simulink model "e8_1_sim"  (R2017b)
settings: Solver=ode4  StartTime=0.0  StopTime=30  FixedStep=0.001  RelTol=1e-3
values from neighbouring files (symbols this model uses):
  DEG2RAD = 0.0174533    [Init_control.m]
  Kd_PITCH_AngleRate = 0.001    [Init_control.m]
  Kd_ROLL_AngleRate = 0.001    [Init_control.m]
  Kd_YAW_AngleRate = 0.00    (= 0)    [Init_control.m]
  Ki_PITCH_AngleRate = 0.02    [Init_control.m]
  Ki_ROLL_AngleRate = 0.02    [Init_control.m]
  Ki_YAW_AngleRate = 0.01    [Init_control.m]
  Kp_PITCH_ANGLE = 6.5    [Init_control.m]
  Kp_PITCH_AngleRate = 0.1    [Init_control.m]
  Kp_ROLL_ANGLE = 6.5    [Init_control.m]
  Kp_ROLL_AngleRate = 0.1    [Init_control.m]
  Kp_YAW_ANGLE = 3    [Init_control.m]
  Kp_YAW_AngleRate = 0.5    [Init_control.m]
  Kpxp = 1.0    (= 1)    [Init_control.m]
  Kpyp = 1.0    (= 1)    [Init_control.m]
  Kpzp = 4.0    (= 4)    [Init_control.m]
  Kvxd = 0.01    [Init_control.m]
  Kvxi = 0.1    [Init_control.m]
  Kvxp = 3.0    (= 3)    [Init_control.m]
  Kvyd = 0.01    [Init_control.m]
  Kvyi = 0.1    [Init_control.m]
  Kvyp = 3.0    (= 3)    [Init_control.m]
  Kvzd = 0.005    [Init_control.m]
  Kvzi = 0.01    [Init_control.m]
  Kvzp = 0.45    [Init_control.m]
  MAX_CONTROL_ANGLE_NAV_PITCH = 15    [Init_control.m]
  MAX_CONTROL_ANGLE_NAV_ROLL = 15    [Init_control.m]
  MAX_CONTROL_ANGLE_PITCH = 35    [Init_control.m]
  MAX_CONTROL_ANGLE_RATE_PITCH = 220    [Init_control.m]
  MAX_CONTROL_ANGLE_RATE_ROLL = 220    [Init_control.m]
  MAX_CONTROL_ANGLE_RATE_Y = 200    [Init_control.m]
  MAX_CONTROL_ANGLE_ROLL = 35    [Init_control.m]
  MAX_CONTROL_VELOCITY_XY = 5    [Init_control.m]
  MAX_CONTROL_VELOCITY_Z = 3    [Init_control.m]
  Saturation_I_ah = 3.43    [Init_control.m]
  Saturation_I_az = 5    [Init_control.m]
  Saturation_I_RP_Max = 0.3    [Init_control.m]
  Saturation_I_RP_Min = -0.3    [Init_control.m]
  Saturation_I_Y_Max = 0.2    [Init_control.m]
  Saturation_I_Y_Min = -0.2    [Init_control.m]
  THR_HOVER = 0.609    [Init_control.m]
undefined symbols (not defined in the file or in its folder): DiscIntNeverNeededParam, earthRadius, KiRollAttitude, ModelInit_AngEuler, ModelInit_PosE, ModelInit_Rads, ModelInit_RateB, ModelInit_VelB, ModelParam_envGravityAcc, ModelParam_motorCr, ModelParam_motorJm, ModelParam_motorT, ModelParam_motorWb, ModelParam_rotorCm, ModelParam_rotorCt, ModelParam_uavCd, ModelParam_uavJ, ModelParam_uavMass, ModelParam_uavR, Receive, Send
libraries: simulink x10, aerolibfltsims x3, sharedutil x2, aerolibanimutils x1
(part 2 of 2)

== matlab function e8_1_sim/Control System/InputConditioning/deadzone2 ==
  data: u input; y output
function y = fcn(u)
%Function description:
%  Control the range of the remote control input from RCMin to RCMax, and set
%  a dead zone with a dead zone size of ±deadZone,the output y is
%  normalized to 0~1.You can get the RC calibration parameters in QGC.
RCMin = 1100;
RCMax = 1900;
RCMid = (RCMin + RCMax)/2;
deadZoneRate = 0.05;
deadZone = deadZoneRate*(RCMax - RCMin);
k = 1/(RCMax - RCMid - deadZone);
%Limiting
if(u < RCMin)
    u = RCMin;
elseif(u > RCMax)
    u = RCMax;
end
%dead zone and normalize
 if(u > RCMid + deadZone)
    y = (u-RCMid - deadZone)*k;
 elseif(u < RCMid - deadZone)
     y = (u - RCMid + deadZone)*k;
 else
     y = 0;
 end

 end

== matlab function e8_1_sim/Control System/Subsystem/AttitudeControl/yawAngle_d/MATLAB Function1 ==
  settings: updateMethod=DISCRETE
  data: yaw input; yaw_rate input; yaw_d output; reset input; timestamp input
function yaw_d  = fcn(yaw, yaw_rate, reset, timestamp)

persistent yaw1;
if isempty(yaw1)
    yaw1 = yaw;
end

persistent timestamp_old;
if isempty(timestamp_old)
    timestamp_old = 0;
end


T = timestamp - timestamp_old;
if T > 0.2
    T = 0.2;
end
if T < 0
    T = 0;
end
if reset
    yaw1 = yaw;
else
   yaw1 = yaw1 + yaw_rate*T;
end

if yaw1 > pi  && yaw < 0
    yaw1 = yaw1- 2*pi;
end
if yaw1 < -pi && yaw > 0
    yaw1 = yaw1 + 2*pi;
end
yaw_d = yaw1;

timestamp_old = timestamp;

== matlab function e8_1_sim/Control System/Subsystem/pwm_out2 ==
  data: Roll input; M1 output; Pitch input; Yaw input; Thrust input; M2 output; M3 output; M4 output
function [M1, M2, M3, M4] = motor_mixer(Roll, Pitch, Yaw, Thrust)
%Function description;
%  Assign the attitude controller output to the motor control. The multi-rotor type is quadrotor-X type,
%  and the propeller serial number is as follows:
%3     1
%  \ /
%  / \
%2     4
%Input：
%  Roll, Pitch, Yaw: Attitude controller output.
%  Thrust

idle_PWM = 1000;
scale = 1000;

M1 = (Thrust - Roll + Pitch + Yaw) * scale + idle_PWM;
M2 = (Thrust + Roll - Pitch + Yaw) * scale + idle_PWM;
M3 = (Thrust + Roll + Pitch - Yaw) * scale + idle_PWM;
M4 = (Thrust - Roll - Pitch - Yaw) * scale + idle_PWM;

== matlab function e8_1_sim/Quadcopter Dynamics/Rigid Model/Calculate the rotation matrix and Euler angle/Quaternion to Euler ==
  data: q input; y output
function y = fcn(q)
 %Function description;
%  Quaternion to Euler
phi = atan2(2*(q(1)*q(2) + q(3)*q(4)), (1 - 2*(q(2)*q(2) + q(3)*q(3))));
theta = asin(2*(q(1)*q(3) - q(2)*q(4)));
psi = atan2(2*(q(1)*q(4) + q(2)*q(3)), (1 - 2*(q(3)*q(3) + q(4)*q(4))));
y = [phi theta psi];

== matlab function e8_1_sim/Quadcopter Dynamics/Rigid Model/Calculate the rotation matrix and Euler angle/Quaternion to rotation matrix ==
  data: q input; Rbe output
function Rbe = fcn(q)
%Function description;
%  The rotation matrix of the body coordinate system to the geodetic coordinate system is obtained from the quaternion
Rbe = [q(1)*q(1) + q(2)*q(2) - q(3)*q(3) - q(4)*q(4), 2*(q(2)*q(3) - q(1)*q(4)), 2*(q(2)*q(4) + q(1)*q(3))
       2*(q(2)*q(3) + q(1)*q(4)), q(1)*q(1) - q(2)*q(2) + q(3)*q(3) - q(4)*q(4), 2*(q(3)*q(4) - q(1)*q(2))
       2*(q(2)*q(4) - q(1)*q(3)), 2*(q(3)*q(4) + q(1)*q(2)), q(1)*q(1) - q(2)*q(2) - q(3)*q(3) + q(4)*q(4)];

== matlab function e8_1_sim/Quadcopter Dynamics/Rigid Model/Calculate the rotation matrix and Euler angle/Euler angle to quaternion ==
  data: EulerAngle input; q output
function q = fcn(EulerAngle)
%Function description;
%  Get quaternion from Euler angle
q0 =  cos(EulerAngle(1)/2)*cos(EulerAngle(2)/2)*cos(EulerAngle(3)/2) + sin(EulerAngle(1)/2)*sin((EulerAngle(2)/2))*sin((EulerAngle(3)/2));
q1 = -sin(EulerAngle(1)/2)*cos(EulerAngle(2)/2)*cos(EulerAngle(3)/2) + cos(EulerAngle(1)/2)*sin((EulerAngle(2)/2))*sin((EulerAngle(3)/2));
q2 = -cos(EulerAngle(1)/2)*sin(EulerAngle(2)/2)*cos(EulerAngle(3)/2) - sin(EulerAngle(1)/2)*cos((EulerAngle(2)/2))*sin((EulerAngle(3)/2));
q3 = -cos(EulerAngle(1)/2)*cos(EulerAngle(2)/2)*sin(EulerAngle(3)/2) + sin(EulerAngle(1)/2)*sin((EulerAngle(2)/2))*cos((EulerAngle(3)/2));
q = [q0 q1 q2 q3]';

== matlab function e8_1_sim/Quadcopter Dynamics/Rigid Model/Calculate the rotation matrix and Euler angle/Quaternions model ==
  data: pqr input; qdot output; q input
function qdot = fcn(pqr, q)
%Function description;
%  Quaternions model
qdot = 0.5*[0, -pqr(1), -pqr(2), -pqr(3); pqr(1), 0, pqr(3), -pqr(2); pqr(2), -pqr(3), 0, pqr(1); pqr(3), pqr(2), -pqr(1), 0]*q;

== matlab function e8_1_sim/Control System/Subsystem/position_control/MATLAB Function ==
  data: eax input; eay input; psi input; phi output; theta output
function [phi, theta] = fcn(eax, eay, psi)
%Function description:
%  Convert the desired horizontal acceleration to the desired attitude angle
%Input:
%  eax, eaxy: desired horizontal acceleration
%  psi: yaw
%Output:
%  phi, theta: desired roll angle and desired pitch angle
g = 9.8;
phi = (-sin(psi)*eax + cos(psi)*eay)/g;
theta = (-cos(psi)*eax - sin(psi)*eay)/g;

== matlab function e8_1_sim/Quadcopter Dynamics/Rigid Model/Rigid-Body Dynamic Model/gyroscopic torques ==
  data: Jrp input; MotorRads input; pqr input; Ga output
function Ga = fcn(Jrp, MotorRads, pqr)
 %Function description;
%  Calculating gyro moment
%Input:
%  Jrp: Moment of inertia of motor rotor + propeller
%  MotorRads: Motor speed,uint:rad/s
%  pqr: Angular velocity in the body coordinate system
Ga = zeros(3,1);
Ga(1) = Jrp*pqr(2)*(-MotorRads(1) - MotorRads(2) + MotorRads(3) + MotorRads(4));
Ga(2) = Jrp*pqr(1)*( MotorRads(1) + MotorRads(2) - MotorRads(3) - MotorRads(4));

== stateflow chart e8_1_sim/Control System/mode switch ==
  state return1
    entry:state=1
  state land
    entry:state=2
  state manual
    entry:state=0
  manual -> return1 [order 1] : [MIE2==2]
  return1 -> manual : [MIE2==1]
  land -> manual : [(MIE2==1)]
  manual -> land [order 2] : [MIE2==3]
  (default) -> manual
  data: state output; MIE2 input

== matlab function e8_1_sim/Control System/InputConditioning/f1 ==
  data: in input; y output; hover input
function y = thr_curve(in, hover)
%Function description:
%  After this function, when the throttle is in the middle position, the output is hovering throttle hover
%Input:
%  in: Throttle normalized value, range (0~1)
%  hover: Hovering throttle value
%Output:
%  Processed throttle value
if in < 0.5
	y=2 * in * hover;
else
	y=hover + 2 * (in - 0.5) * (1.0 - hover);
end

== matlab function e8_1_sim/Control System/MATLAB Function2 ==
  data: ch5 input; MIE2 output
function MIE2 = fcn(ch5)
%Function description:
%  Map the remote CH5 channel to manual operation instructions
%Input:
%  ch5: Remote control CH5 channel input
%Output:
%  MIE2:Manual operation instruction
%  1: MANUAL FLIGHT MODE
%  2: RTL MODE
%  3: AUTO-LANDING MODE
if ch5 < 1400
    MIE2 = int8(1);
elseif ch5 < 1600
    MIE2 = int8(2);
else
    MIE2 = int8(3);
end

== matlab function e8_1_sim/Control System/MATLAB Function1 ==
  settings: updateMethod=DISCRETE
  data: state input; vxd output; vyd output; vzd output; x input; y input; z input; vx input; vy input; vz input; xd output; yd output; zd output
function [vxd, vyd, vzd, xd, yd, zd] = fcn(state, x, y, z, vx, vy, vz)
%Function description:
%  Flight mode switch  implemention.
%Input:
%  state: flight mode
%  x, y, z: current position
%  vx, vy,vz: current velocity
%Output:
%  vx_d, vy_d, vz_d: desired velocity
%  x_d, y_d, z_d: desired position
persistent hold_x_flag;
if isempty(hold_x_flag)
    hold_x_flag = 0;
end
persistent hold_y_flag;
if isempty(hold_y_flag)
    hold_y_flag = 0;
end
persistent hold_z_flag;
if isempty(hold_z_flag)
    hold_z_flag = 0;
end
persistent x1;
if isempty(x1)
    x1 = 0;
end
persistent y1;
if isempty(y1)
    y1 = 0;
end

persistent z1;
if isempty(z1)
    z1 = 0;
end

heightSafe = 50;  % expected height is set to 50 m
if state == 1  %Return, the altitude below the specified threshold, first rise to the specified value
    vxd = 0;  %Reduce the horizontal speed to 0
    vyd = 0;
    hold_x_flag = 0;
    hold_y_flag = 0;
    if abs(z) < heightSafe
        z1 = -heightSafe; vzd = 0; 
        hold_z_flag = 0;
    else
        vzd = 0;
        if abs(vz) < 6 &&(hold_z_flag < 0.5)
            z1 = z; 
            hold_z_flag = 1;
        end
        if ~(abs(vz) < 6)
           z1 = z;
           hold_z_flag = 0;
        end
    end
    
    if abs(vx) < 8
       x1 = 0; 
   end
   if ~(abs(vx) < 8)
       x1 = x; 
   end
   if abs(vy) < 8 
       y1 = 0;
   end
   if ~(abs(vy) < 8)
       y1 = y;
   end
elseif state == 2  %land
    vxd = 0; vyd = 0;
   z1 = 0; vzd = 0;  %desired height is 0,land
   hold_z_flag = 0;
   %olve the drift problem
   if abs(vx) < 8 && (hold_x_flag < 0.5)
       x1 = x; 
       hold_x_flag = 1;
   end
   if ~(abs(vx) < 8)
       x1 = x; 
       hold_x_flag = 0;
   end
   if abs(vy) < 8 && (hold_y_flag < 0.5)
       y1 = y;
       hold_y_flag = 1;
   end
   if ~(abs(vy) < 8)
       y1 = y;
       hold_y_flag = 0;
   end
   
else %mannual control mode
   x1 = x; vxd = 0;
   y1 = y; vyd = 0;
   z1 = z; vzd = 0;
   
   hold_x_flag = 0;
   hold_y_flag = 0;
   hold_z_flag = 0;
end

 xd = x1;
 yd = y1;
 zd = z1;
